simulink model "project_model"  (R2020b)
settings: Solver=VariableStepAuto  StartTime=0.0  StopTime=10.0  RelTol=1e-3
settings Model: Creator=ASUS  LastModifiedBy=ASUS

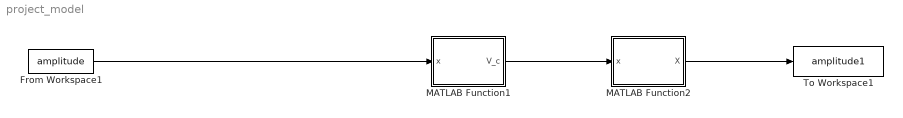
== system project_model ==
  From Workspace1 : FromWorkspace  VariableName=amplitude
  MATLAB Function1 : MATLAB Function  TreatAsAtomicUnit=on
  MATLAB Function2 : MATLAB Function  TreatAsAtomicUnit=on
  To Workspace1 : ToWorkspace  VariableName=amplitude1  SaveFormat=Timeseries  SampleTime=-1
  wires:
  From Workspace1/1 -> MATLAB Function1/1(x)
  MATLAB Function1/1(V_c) -> MATLAB Function2/1(x)
  MATLAB Function2/1(X) -> To Workspace1/1

== matlab function project_model/MATLAB Function2 ==
  data: x input; X output
function X = fcn(x)
    coder.extrinsic("lowPassFilter");
    X = double(0);
    X = double(lowPassFilter(x));
end

== matlab function project_model/MATLAB Function1 ==
  data: x input; V_c output
function V_c = fcn(x)
    g=0.013;
    m = length(x);
    V_c = x;
    for i=1:m-1
        if(x(i+1)>V_c(i))
            V_c(i+1) = x(i+1);
        else
            V_c(i+1) = V_c(i) - g*V_c(i);
        end
    end
end
